simulink model "Assem_for_matlab"  (R2024a)
settings: Solver=VariableStepAuto  StartTime=0.0  StopTime=5  RelTol=1e-3
model workspace: external: MATLAB File F:\Graduation_Project\Code_Cpp\Delta_Robot_v2\Matlab_Simscape_Multibody\Assem_for_matlab_DataFile.m (data not in the file)
undefined symbols (not defined in the file or in its folder): smiData, X, Y, Z
libraries: sm_lib x144, nesl_utility x7, simulink_extras x4
(part 1 of 4)
settings Model: Creator=ACER  LastModifiedBy=ACER

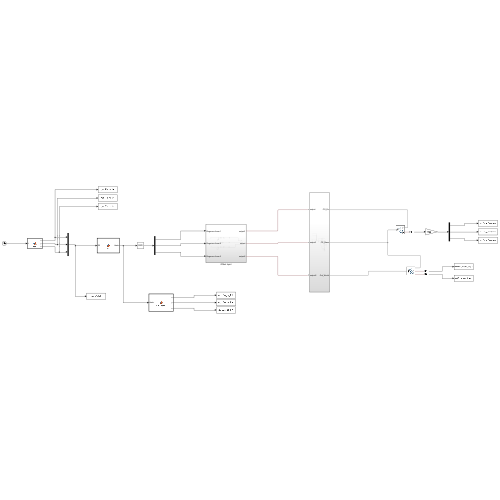
[thumbnail: Simulink's stored preview of the top-level diagram]
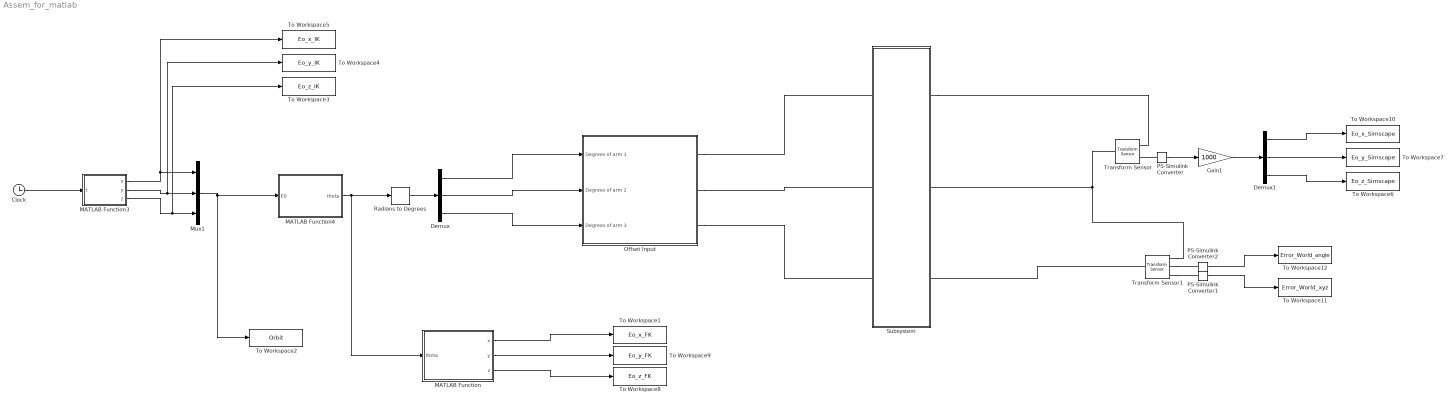
== system Assem_for_matlab ==
  Clock : Clock
  Demux : Demux  Outputs=3
  Demux1 : Demux  Outputs=3
  Gain1 : Gain  Gain=1000
  MATLAB Function : MATLAB Function  TreatAsAtomicUnit=on
  MATLAB Function3 : MATLAB Function  TreatAsAtomicUnit=on
  MATLAB Function4 : MATLAB Function  TreatAsAtomicUnit=on
  Mux1 : Mux  Inputs=3
  "Offset Input " : Subsystem
  PS-Simulink Converter : nesl_utility/PS-Simulink Converter  PhysicalDomain=network_engine_domain  SubClassName=ps_output  LeftPortType=input  RightPortType=output  PseudoPeriodic=off  Frequencies=[]  VectorFormat=inherit  Unit=inherit  AffineConversion=off
  PS-Simulink Converter1 : nesl_utility/PS-Simulink Converter  PhysicalDomain=network_engine_domain  SubClassName=ps_output  LeftPortType=input  RightPortType=output  PseudoPeriodic=off  Frequencies=[]  VectorFormat=inherit  Unit=inherit  AffineConversion=off
  PS-Simulink Converter2 : nesl_utility/PS-Simulink Converter  PhysicalDomain=network_engine_domain  SubClassName=ps_output  LeftPortType=input  RightPortType=output  PseudoPeriodic=off  Frequencies=[]  VectorFormat=inherit  Unit=inherit  AffineConversion=off
  Radians to Degrees : simulink_extras/Transformations/Radians to Degrees
  Subsystem : Subsystem
  To Workspace1 : ToWorkspace  VariableName=Eo_x_FK  SaveFormat=Timeseries  SampleTime=-1
  To Workspace10 : ToWorkspace  VariableName=Eo_x_Simscape  SaveFormat=Timeseries  SampleTime=-1
  To Workspace11 : ToWorkspace  VariableName=Error_World_xyz  SaveFormat=Timeseries  SampleTime=-1
  To Workspace12 : ToWorkspace  VariableName=Error_World_angle  SaveFormat=Timeseries  SampleTime=-1
  To Workspace2 : ToWorkspace  VariableName=Orbit  SampleTime=-1
  To Workspace3 : ToWorkspace  VariableName=Eo_z_IK  SaveFormat=Timeseries  SampleTime=-1
  To Workspace4 : ToWorkspace  VariableName=Eo_y_IK  SaveFormat=Timeseries  SampleTime=-1
  To Workspace5 : ToWorkspace  VariableName=Eo_x_IK  SaveFormat=Timeseries  SampleTime=-1
  To Workspace6 : ToWorkspace  VariableName=Eo_z_Simscape  SaveFormat=Timeseries  SampleTime=-1
  To Workspace7 : ToWorkspace  VariableName=Eo_y_Simscape  SaveFormat=Timeseries  SampleTime=-1
  To Workspace8 : ToWorkspace  VariableName=Eo_z_FK  SaveFormat=Timeseries  SampleTime=-1
  To Workspace9 : ToWorkspace  VariableName=Eo_y_FK  SaveFormat=Timeseries  SampleTime=-1
  Transform Sensor : sm_lib/Frames and Transforms/Transform Sensor  MeasurementFrame=World  RotationSequence=XYX  SenseAngle=off  SenseAxis=off  SenseQ=off  SenseR=off  SenseRotationSequence=off  SenseOmegaX=off  SenseOmegaY=off  SenseOmegaZ=off  SenseOmega=off  SenseQDot=off  SenseRDot=off  SenseRotationSequenceDot=off  SenseAlphaX=off  SenseAlphaY=off  SenseAlphaZ=off  SenseAlpha=off  SenseQDDot=off  SenseRDDot=off  SenseX=off  SenseY=off  SenseZ=off  SenseXYZ=on  SenseRad=off  SenseAzim=off  SenseDist=off  SenseInc=off  SenseXDot=off  SenseYDot=off  SenseZDot=off  SenseXYZDot=off  SenseRadDot=off  SenseAzimDot=off  SenseDistDot=off  SenseIncDot=off  SenseXDDot=off  SenseYDDot=off  SenseZDDot=off  SenseXYZDDot=off  SenseRadDDot=off  SenseAzimDDot=off  SenseDistDDot=off  SenseIncDDot=off
  Transform Sensor1 : sm_lib/Frames and Transforms/Transform Sensor  MeasurementFrame=World  RotationSequence=XYX  SenseAngle=on  SenseAxis=off  SenseQ=off  SenseR=off  SenseRotationSequence=off  SenseOmegaX=off  SenseOmegaY=off  SenseOmegaZ=off  SenseOmega=off  SenseQDot=off  SenseRDot=off  SenseRotationSequenceDot=off  SenseAlphaX=off  SenseAlphaY=off  SenseAlphaZ=off  SenseAlpha=off  SenseQDDot=off  SenseRDDot=off  SenseX=off  SenseY=off  SenseZ=off  SenseXYZ=on  SenseRad=off  SenseAzim=off  SenseDist=off  SenseInc=off  SenseXDot=off  SenseYDot=off  SenseZDot=off  SenseXYZDot=off  SenseRadDot=off  SenseAzimDot=off  SenseDistDot=off  SenseIncDot=off  SenseXDDot=off  SenseYDDot=off  SenseZDDot=off  SenseXYZDDot=off  SenseRadDDot=off  SenseAzimDDot=off  SenseDistDDot=off  SenseIncDDot=off
  wires:
  PS-Simulink Converter1/1 -> To Workspace11/1
  PS-Simulink Converter2/1 -> To Workspace12/1
  PS-Simulink Converter/1 -> Gain1/1
  Gain1/1 -> Demux1/1
  Demux1/2 -> To Workspace7/1
  Demux1/1 -> To Workspace10/1
  Demux1/3 -> To Workspace6/1
  MATLAB Function/3(z) -> To Workspace8/1
  MATLAB Function/1(x) -> To Workspace1/1
  Mux1/1 -> To Workspace2/1, MATLAB Function4/1(E0)
  MATLAB Function/2(y) -> To Workspace9/1
  MATLAB Function3/1(x) -> Mux1/1, To Workspace5/1
  MATLAB Function3/3(z) -> To Workspace3/1, Mux1/3
  Clock/1 -> MATLAB Function3/1(t)
  MATLAB Function4/1(theta) -> MATLAB Function/1(theta), Radians to Degrees/1
  Radians to Degrees/1 -> Demux/1
  MATLAB Function3/2(y) -> Mux1/2, To Workspace4/1
  Demux/1 -> "Offset Input "/1(Degrees of arm 1)
  Demux/2 -> "Offset Input "/2(Degrees of arm 2)
  Demux/3 -> "Offset Input "/3(Degrees of arm 3)
  connections:
  Transform Sensor1/RConn1 -- Transform Sensor/LConn1 -- Subsystem/RConn2
  Transform Sensor1/RConn2 -- PS-Simulink Converter2/LConn1
  Transform Sensor1/LConn1 -- Subsystem/RConn3
  Transform Sensor1/RConn3 -- PS-Simulink Converter1/LConn1
  PS-Simulink Converter/LConn1 -- Transform Sensor/RConn2
  Subsystem/RConn1 -- Transform Sensor/RConn1
  "Offset Input "/RConn3 -- Subsystem/LConn3
  "Offset Input "/RConn2 -- Subsystem/LConn2
  "Offset Input "/RConn1 -- Subsystem/LConn1

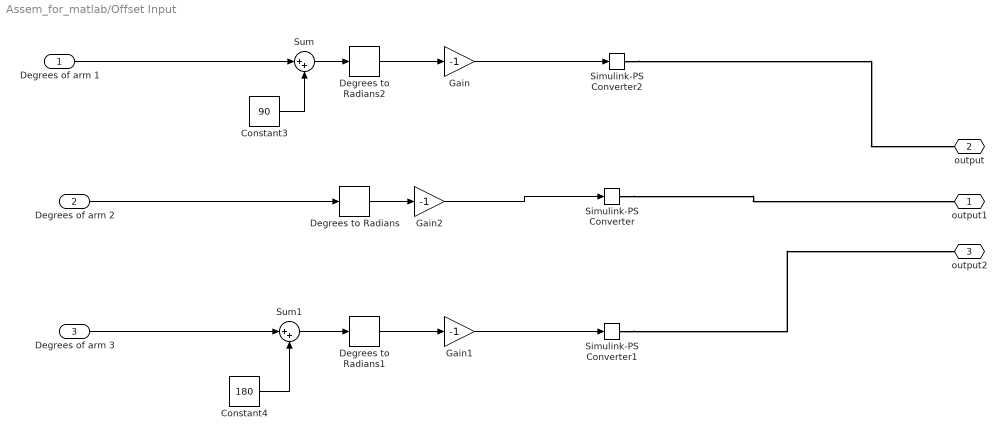
== system Assem_for_matlab/Offset Input  ==
  Degrees of arm 1 : Inport
  Degrees of arm 2 : Inport  Port=2
  Degrees of arm 3 : Inport  Port=3
  Constant3 : Constant  Value=90
  Constant4 : Constant  Value=180
  Degrees to Radians : simulink_extras/Transformations/Degrees to Radians
  Degrees to Radians1 : simulink_extras/Transformations/Degrees to Radians
  Degrees to Radians2 : simulink_extras/Transformations/Degrees to Radians
  Gain : Gain  Gain=-1
  Gain1 : Gain  Gain=-1
  Gain2 : Gain  Gain=-1
  Simulink-PS Converter : nesl_utility/Simulink-PS Converter  PhysicalDomain=network_engine_domain  SubClassName=ps_input  LeftPortType=input  RightPortType=output  PseudoPeriodic=off  Frequencies=[]  NoiseDistribution=none  NoiseParameters=[]  Unit=1  AffineConversion=off  FilteringAndDerivatives=zero  SimscapeFilterOrder=2  InputFilterTimeConstant=0.01  UdotUserProvided=0
  Simulink-PS Converter1 : nesl_utility/Simulink-PS Converter  PhysicalDomain=network_engine_domain  SubClassName=ps_input  LeftPortType=input  RightPortType=output  PseudoPeriodic=off  Frequencies=[]  NoiseDistribution=none  NoiseParameters=[]  Unit=1  AffineConversion=off  FilteringAndDerivatives=zero  SimscapeFilterOrder=2  InputFilterTimeConstant=0.01  UdotUserProvided=0
  Simulink-PS Converter2 : nesl_utility/Simulink-PS Converter  PhysicalDomain=network_engine_domain  SubClassName=ps_input  LeftPortType=input  RightPortType=output  PseudoPeriodic=off  Frequencies=[]  NoiseDistribution=none  NoiseParameters=[]  Unit=1  AffineConversion=off  FilteringAndDerivatives=zero  SimscapeFilterOrder=2  InputFilterTimeConstant=0.01  UdotUserProvided=0
  Sum : Sum  Inputs=|++
  Sum1 : Sum  Inputs=|++
  output1 : PMIOPort  Side=Right
  output : PMIOPort  Port=2  Side=Right
  output2 : PMIOPort  Port=3  Side=Right
  wires:
  Degrees to Radians/1 -> Gain2/1
  Degrees to Radians2/1 -> Gain/1
  Sum1/1 -> Degrees to Radians1/1
  Degrees to Radians1/1 -> Gain1/1
  Constant4/1 -> Sum1/2
  Sum/1 -> Degrees to Radians2/1
  Constant3/1 -> Sum/2
  Degrees of arm 3/1 -> Sum1/1
  Degrees of arm 1/1 -> Sum/1
  Degrees of arm 2/1 -> Degrees to Radians/1
  Gain/1 -> Simulink-PS Converter2/1
  Gain1/1 -> Simulink-PS Converter1/1
  Gain2/1 -> Simulink-PS Converter/1
  connections:
  Simulink-PS Converter/RConn1 -- output1/RConn1
  Simulink-PS Converter2/RConn1 -- output/RConn1
  Simulink-PS Converter1/RConn1 -- output2/RConn1
